simulink model "gene_traj"  (R2017a)
settings: Solver=VariableStepAuto  StartTime=0.0  StopTime=100.0  RelTol=1e-3
values from neighbouring files (symbols this model uses):
  P = 0.5    [robot.m]
  R = 0.5    [robot.m]
  w = 0.5    [robot.m]
  x0 = 1    [robot.m]
  y0 = L2    (= 1)    [robot.m]
  z0 = L1    (= 0.5)    [robot.m]
settings Model: Creator=massona  LastModifiedBy=massona
settings DataIOCC: Refine=100

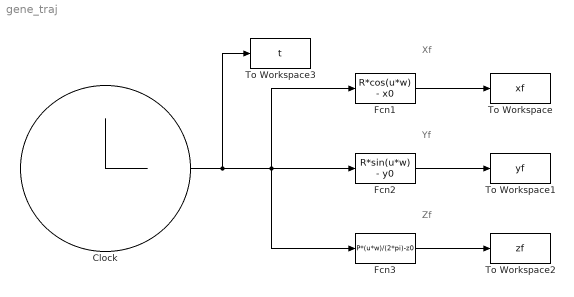
== system gene_traj ==
  note: Xf
  note: Yf
  note: Zf
  Clock : Clock
      settings: Decimation=100
  Fcn1 : Fcn  Expr=R*cos(u*w) - x0
  Fcn2 : Fcn  Expr=R*sin(u*w) - y0
  Fcn3 : Fcn  Expr=P*(u*w)/(2*pi)-z0
  To Workspace : ToWorkspace  VariableName=xf  SampleTime=-1
  To Workspace1 : ToWorkspace  VariableName=yf  SampleTime=-1
  To Workspace2 : ToWorkspace  VariableName=zf  SampleTime=-1
  To Workspace3 : ToWorkspace  VariableName=t  SampleTime=-1
  wires:
  Fcn1/1 -> To Workspace/1
  Fcn2/1 -> To Workspace1/1
  Fcn3/1 -> To Workspace2/1
  Clock/1 -> To Workspace3/1, Fcn3/1, Fcn1/1, Fcn2/1
